simulink model "displayTest"  (R2022b)
settings: Solver=FixedStepDiscrete  StartTime=0.0  StopTime=10.0  FixedStep=0.01  RelTol=1e-3  EnableMultiTasking=on
PreLoadFcn:
  | try, model_open; catch, disp('Error occurred while executing model pre-load callback: model_open.m'); disp('Please assure that the MATLAB working directory is set to the model directory before opening.'); end
InitFcn:
  | try, model_open; catch, end
model workspace (MAT data in the model file):
  IOScreen_Label_XCoord = 1
  IOScreen_Row1_YCoord = 1
  IOScreen_Row2_YCoord = 12
  IOScreen_Value_XCoord = 110
  MainScreen_Row1_YCoord = 7
  MainScreen_Row2_YCoord = 23
  MainScreen_Symbols_XCoord = 1
  MainScreen_Units_XCoord = 69
  MainScreen_Value_XCoord = 64
undefined symbols (not defined in the file or in its folder): curr_screen, DISP, gesture, raptor_get_buildNum, raptor_get_safe_string, raptor_hwexp, raptor_xcp_function, Screens, VC500
libraries: Raptor_display_lib x93, Raptor_lib x40, Raptor_Datalogging_lib x10, simulink_extras x3, simulink x2
(part 1 of 3)
CloseFcn:
  | try, model_close; catch, end
settings Model: Raptor_Target=DISP-VC500-1904  RaptorUIDSize=4  Raptor_Calloc=NonVolatile (EEPROM)  RaptorBuildNum=0  Raptor_ecuaddr=253  Raptor_IsLiteMode=0  SimulationMode=rapid-accelerator  Creator=Ben  LastModifiedBy=Jhon
settings SolverCC: AlgebraicLoopSolver=TrustRegion
settings DataIOCC: LimitDataPoints=on  SaveFormat=Array  SignalLoggingSaveFormat=ModelDataLogs  ReturnWorkspaceOutputs=off
settings OptimizationCC: DefaultParameterBehavior=Inlined  ExpressionDepthLimit=2147483647  InitFltsAndDblsToZero=on  LifeSpan=1  EfficientTunableParamExpr=on
settings DebuggingCC: CheckSSInitialOutputMsg=off  SolverPrmCheckMsg=warning  InheritedTsInSrcMsg=none  FcnCallInpInsideContextMsg=warning  UnconnectedInputMsg=warning  UnconnectedOutputMsg=warning  UnconnectedLineMsg=warning  StateNameClashWarn=warning  PregeneratedLibrarySubsystemCodeDiagnostic=none  SFUnexpectedBacktrackingDiag=warning  SFNoUnconditionalDefaultTransitionDiag=warning  SFExecutionAtInitializationDiag=none  SFMachineParentedDataDiag=warning  ArithmeticOperatorsInVariantConditions=warning
settings HardwareCC: ProdBitPerPointer=32  ProdBitPerSizeT=32  ProdBitPerPtrDiffT=32  ProdLargestAtomicInteger=Long  ProdWordSize=32  ProdHWDeviceType=ARM Compatible->ARM 9  TargetIntDivRoundTo=Zero  TargetEndianess=BigEndian  ProdEqTarget=off
settings ModelReferenceCC: EnableRefExpFcnMdlSchedulingChecks=on  PropagateSignalLabelsOutOfModel=off
settings SFSimCC: SimUseLocalCustomCode=off  MATLABDynamicMemAlloc=off  CustomCodeUndefinedFunction=UseInterfaceOnly
settings RTWCC: Description=Raptor (tm)  SystemTargetFile=raptor.tlc  GenCodeOnly=on  MakeCommand=raptor_make_rtw  TemplateMakefile=raptor.tmf  RTWUseLocalCustomCode=off
settings CodeAppCC: IgnoreCustomStorageClasses=off  MaxIdLength=100  CustomSymbolStrType=$N$R$M  StateflowObjectComments=on  InternalIdentifier=Classic
settings STFCustomTargetCC: GenerateSampleERTMain=on  ModelReferenceCompliant=off  CombineOutputUpdateFcns=on  ERTCustomFileBanners=on  SupportContinuousTime=off  SupportNonInlinedSFcns=off  RemoveResetFunc=on  MATLABClassNameForMDSCustomization=Simulink.SoftwareTarget.ERTCustomization  SystemTargetFile=raptor.tlc
settings ERTTargetCC: MultiwordLength=2048  GenerateSampleERTMain=on  ModelReferenceCompliant=off  ParMdlRefBuildCompliant=off  CompOptLevelCompliant=off  ConcurrentExecutionCompliant=off  ModelStepFunctionPrototypeControlCompliant=off  CPPClassGenCompliant=off  UseToolchainInfoCompliant=off  ExtModeMexFile=noextcomm  InlinedParameterPlacement=NonHierarchical  ERTCustomFileTemplate=example_file_process.tlc  ConvertIfToSwitch=off  SuppressUnreachableDefaultCases=off
settings ConfigComp: CovMetricSettings=dw  CovSaveCumulativeToWorkspaceVar=on  CovSaveSingleToWorkspaceVar=on  CovExternalEMLEnable=off

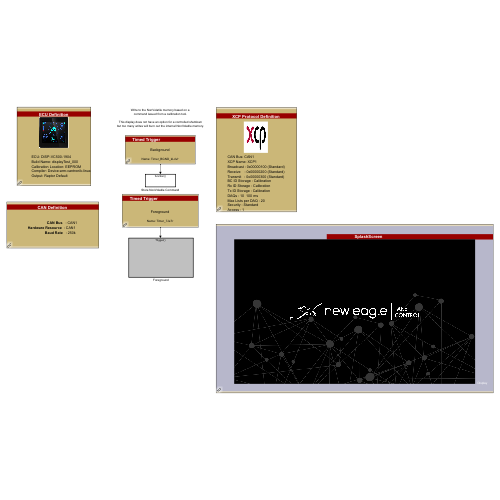
[thumbnail: Simulink's stored preview of the top-level diagram]
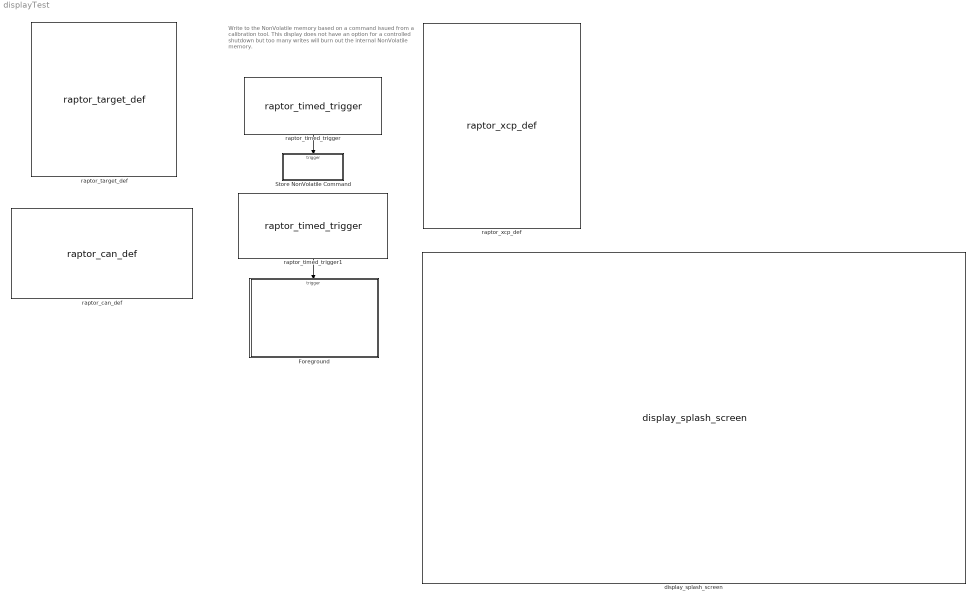
== system displayTest ==
  note: Write to the NonVolatile memory based on a
      | command issued from a calibration tool.
      |
      | This display does not have an option for a controlled shutdown
      | but too many writes will burn out the internal NonVolatile memory.
  Foreground : Subsystem
  Store NonVolatile Command : Subsystem  TreatAsAtomicUnit=on
  display_splash_screen : Raptor_display_lib/Screen Functions/display_splash_screen  ImageFile=background_newsplash.bmp
      settings: SourceProductName=Raptor Display Library
  raptor_can_def : Raptor_lib/CAN/raptor_can_def  canBus='CAN1'  resourceValues=CAN1|(None)  resource=CAN1  baudRateValues=125k|250k|500k|1000k  baudRate=250k  enable_baud_rate_config=0  sim_func_name='ConfigureCANBaudRate'  createButton=[]  txQueueSize=16  rxQueueSize=16
      settings: SourceProductName=Raptor
  raptor_target_def : Raptor_lib/Configuration/raptor_target_def  targetValues=BCM-5646-48-1404|CSM-S32K148-030-1903|DISP-VC128-1901|DISP-VC320L-1402|DISP-VC320-1204|DISP-VC800-1402|DISP-VC500-1904|DISP-VC700-2003|DISP-VC300R-2004|GCM-5634M-070-1459|GCM-5634M-070-1559|GCM-5634M-070-1562|ECM-1793-196-1503|GCM-1793-196-1503|GCM-5605B-048-1906|GCM-5607B-80-1901|GCM-5607B-80-1903|GCM-5607B-80-2001|GCM-5746R-048-1902|HCM-5534-50-1203|HCM-5534-90-1201|HCM-5534-90-1302|HCM-5534-90-1601|HCM-5534-90-1602|HCM-5604-36-1303|HCM-5604-36-1702|HCM-ARM4-070-1401|HCM-ARM4-070-1601|UAS-564A-WAL  target=DISP-VC500-1904  simpack=0  simulator=0  heap=2*1024  stack=2*1024  fgndStack=2*1024  bgndStack=2*1024  idleStack=1024  intStack=1536  sdStack=1024  appStack=1024  ecuaddr=253  uds_server_addr_ext=0  uds_server_addr=hex2dec('600')  uds_client_addr=hex2dec('650')  callocValues=Constant (FLASH)|NonVolatile (EEPROM)  calloc=NonVolatile (EEPROM)  compilerValues=Device:arm-cantronik-linux-gnueabihf_5.4.2 Simulator:None (disabled)|Device:arm-cantronik-linux-gnueabihf_5.4.2 Simulator:Visual Studio Community 2017  compiler=Device:arm-cantronik-linux-gnueabihf_5.4.2 Simulator:Visual Studio Community 2017  setFileName=1  exeName=[raptor_get_safe_string(bdroot) '_']  addBuildNum=1  minVerChars=3  extraOutput=0  buildLocationValues=Raptor Default|Model Directory|User Defined  buildLocation=Raptor Default  exeLocation=''  exeFileButton=[]  a2lLocation=''  a2lFileButton=[]  rpgLocation=''  rpgFileButton=[]
      settings: SourceProductName=Raptor
  raptor_timed_trigger : Raptor_lib/Triggers/raptor_timed_trigger  triggerValues=Foreground|Foregroundx2|Foregroundx5|Foregroundx10|Foregroundx50|Background|Backgroundx2|Backgroundx5|Backgroundx10|Backgroundx20|Second|Minute  trigger=Background  inherited=0  alwaysEnabled=1  triggerPriority=0  triggerName=BGND_kLoVr
      settings: SourceProductName=Raptor
  raptor_timed_trigger1 : Raptor_lib/Triggers/raptor_timed_trigger  triggerValues=Foreground|Foregroundx5|Foregroundx10|Foregroundx50|Second|Minute  trigger=Foreground  inherited=0  alwaysEnabled=1  triggerPriority=0  triggerName=7Je7r
      settings: SourceProductName=Raptor
  raptor_xcp_def : Raptor_lib/Configuration/raptor_xcp_def  XCPname='XCP1'  canBus='CAN1'  bcID=hex2dec('100')  bcID_TypeValues=Standard|Extended  bcID_Type=Standard  rxID=hex2dec('200')  rxID_TypeValues=Standard|Extended  rxID_Type=Standard  txID=hex2dec('300')  txID_TypeValues=Standard|Extended  txID_Type=Standard  daqRates=[10 100]  numODTs=20  genCANAPE=0  genVISION=0  securityValues=Standard|None|Custom User Defined|MH_SB_4  security=Standard  dllName=raptor_XCPSecurity.dll  accessValues=4|3|2|1  access=1  bcStorageValues=[]  bcStorage=Calibration  txStorageValues=[]  txStorage=Calibration  rxStorageValues=[]  rxStorage=Calibration
      settings: SourceProductName=Raptor
  wires:
  raptor_timed_trigger1/1 -> Foreground/Trigger
  raptor_timed_trigger/1 -> Store NonVolatile Command/Trigger

== system displayTest/Foreground ==
  Trigger : TriggerPort  TriggerType=function-call  VariantControl=Variant  PortDimensions=1
  Display : Subsystem
      mask Display: image(imread('DISP-VC500-1904.jpg'))
  Plant : Subsystem
      mask Display:
      | block = gcb;
      | pos = get_param(gcb, 'Position');
      | 
      | info = imfinfo('VeeCAN500_pinout.png');
      | 
      | pos(3) = pos(1)+info.Width;
      | pos(4) = pos(2)+info.Height;
      | 
      | set_param(block, 'Position', pos);
      | 
      | image(imread('VeeCAN500_pinout.png'));
  wires:
  Display/1(Actuators) -> Plant/1(Actuators)
  Plant/1(Sensors) -> Display/1(Sensors)

== system displayTest/Store NonVolatile Command ==
  note: Setting the StoreNonvolatileCommand value to to 1
      | in the calibration tool will cause this subsystem to execute, calling the 'Store Nonvolatile' function.
      |
      | The StoreNonvolatileCommand value will be set to 0 inside
      | the subsytem so that the Store event happens once.
  function : TriggerPort  TriggerType=function-call  VariantControl=Variant
  Store NV : Subsystem  TreatAsAtomicUnit=on
  raptor_data_def : Raptor_lib/Data Storage/raptor_data_def  dataName='StoreNonVolatileCommand'  initValue=false  dataType=boolean  storage=Volatile (RAM)  calVisible=on  calType=Adjustment  calDispType=Enumeration  calEnum={'Not Writing', 'Start Write'}  calGain=1.0  calOffset=0  calMin=-inf  calMax=inf  calFormat='-1'  calUnit=''  calHelp=''  calAccess=1  calFunction=raptor_xcp_function(gcb)  calDispHeaders=off  calColHeaders={'Col1' 'Col2' 'Col3'}  calRowHeaders={'Row1' 'Row2' 'Row3'}
      settings: SourceProductName=Raptor
  raptor_data_read : Raptor_lib/Data Storage/raptor_data_read  dataName='StoreNonVolatileCommand'  dataShape=Scalar  idxSource=Input  idxRow=1  idxCol=1
      settings: SourceProductName=Raptor
  wires:
  raptor_data_read/1 -> Store NV/Enable

== system displayTest/Foreground/Display ==
  Sensors : Inport
  Data Logging : Subsystem
  Screens : Subsystem
  Unit Delay : UnitDelay  SampleTime=-1  HasFrameUpgradeWarning=on
  Actuators : Outport  VectorParamsAs1DForOutWhenUnconnected=off
  wires:
  Sensors/1 -> Data Logging/2(Sensors), Screens/1(Sensors)
  Screens/1(ActuatorCommands) -> Actuators/1
  Screens/2(DataLogCommands) -> Data Logging/1(Commands)
  Data Logging/1(DataLogState) -> Unit Delay/1
  Unit Delay/1 -> Screens/2(DataLogState)

== system displayTest/Foreground/Plant ==
  Actuators : Inport
  Inputs : Subsystem
  Outputs : Subsystem
  Sensors : Outport  VectorParamsAs1DForOutWhenUnconnected=off
  wires:
  Actuators/1 -> Outputs/1(Commands)
  Inputs/1(Sensors) -> Sensors/1

== system displayTest/Store NonVolatile Command/Store NV ==
  Enable : EnablePort
  Constant : Constant  Value=false
  Function-Call Generator : simulink/Ports & Subsystems/Function-Call Generator  sample_time=-1  numberOfIterations=1  DisallowWideOutput=off
  raptor_data_write : Raptor_lib/Data Storage/raptor_data_write  dataName='StoreNonVolatileCommand'  dataShape=Scalar  idxSource=Input Port  idxRow=1  idxCol=1
      settings: SourceProductName=Raptor
  raptor_store_nv : Raptor_lib/Data Storage/raptor_store_nv  null=0
      settings: SourceProductName=Raptor
  wires:
  Function-Call Generator/1 -> raptor_store_nv/Trigger
  Constant/1 -> raptor_data_write/1

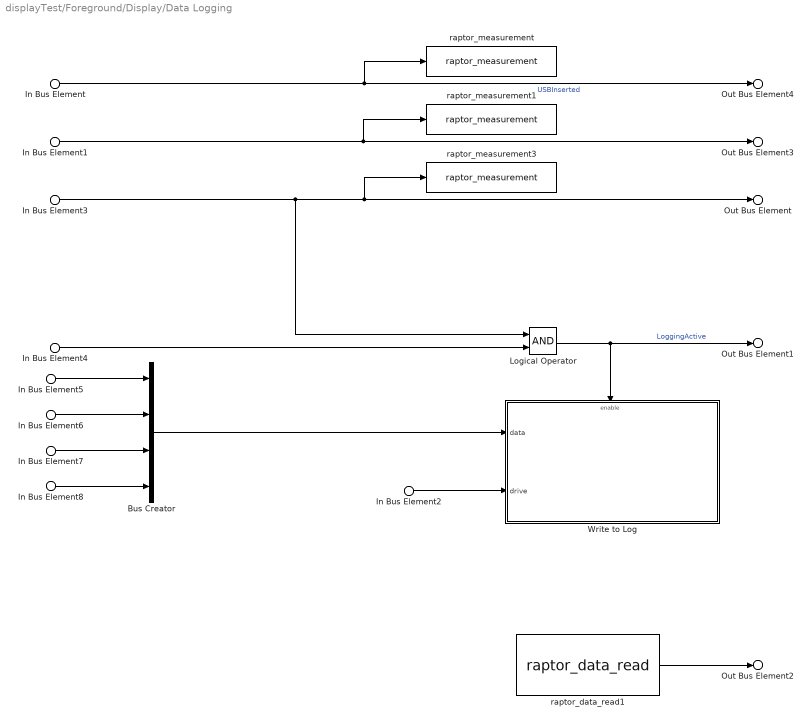
== system displayTest/Foreground/Display/Data Logging ==
  In Bus Element4 : Inport  PortName=Commands  Element=LoggingEnabled
  In Bus Element : Inport  Port=2  PortName=Sensors  Element=USBInserted
  In Bus Element1 : Inport  Port=2  PortName=Sensors  Element=USBEjectReady
  In Bus Element2 : Inport  Port=2  PortName=Sensors  Element=USBPath
  In Bus Element3 : Inport  Port=2  PortName=Sensors  Element=USBReadyToLog
  In Bus Element5 : Inport  Port=2  PortName=Sensors  Element=EngineRPM
  In Bus Element6 : Inport  Port=2  PortName=Sensors  Element=EngineRPMValid
  In Bus Element7 : Inport  Port=2  PortName=Sensors  Element=Illumination
  In Bus Element8 : Inport  Port=2  PortName=Sensors  Element=IlluminationValid
  Bus Creator : BusCreator  Inputs=4
  Logical Operator : Logic  AllPortsSameDT=off  OutDataTypeStr=boolean
  Write to Log : Subsystem
  raptor_data_read1 : Raptor_lib/Data Storage/raptor_data_read  dataName='LogCounter'  dataShape=Scalar  idxSource=Input  idxRow=1  idxCol=1
      settings: SourceProductName=Raptor
  raptor_measurement : Raptor_lib/Data Storage/raptor_measurement  paramName='USBInserted'  nameSource=Parameter  calDispType=Number  calEnum={'False', 'True'}  calGain=1.0  calOffset=0.0  calMax=inf  calMin=-inf  calFormat='-1'  calUnit=''  calHelp=''  calAccess=1  calFunction=raptor_xcp_function(gcb)  calVisible=on
      settings: SourceProductName=Raptor
  raptor_measurement1 : Raptor_lib/Data Storage/raptor_measurement  paramName='EjectReady'  nameSource=Parameter  calDispType=Number  calEnum={'False', 'True'}  calGain=1.0  calOffset=0.0  calMax=inf  calMin=-inf  calFormat='-1'  calUnit=''  calHelp=''  calAccess=1  calFunction=raptor_xcp_function(gcb)  calVisible=on
      settings: SourceProductName=Raptor
  raptor_measurement3 : Raptor_lib/Data Storage/raptor_measurement  paramName='LoggingReady'  nameSource=Parameter  calDispType=Number  calEnum={'False', 'True'}  calGain=1.0  calOffset=0.0  calMax=inf  calMin=-inf  calFormat='-1'  calUnit=''  calHelp=''  calAccess=1  calFunction=raptor_xcp_function(gcb)  calVisible=on
      settings: SourceProductName=Raptor
  Out Bus Element : Outport  VectorParamsAs1DForOutWhenUnconnected=off  PortName=DataLogState  Element=LoggingPossible
  Out Bus Element1 : Outport  VectorParamsAs1DForOutWhenUnconnected=off  PortName=DataLogState  Element=LoggingActive
  Out Bus Element2 : Outport  VectorParamsAs1DForOutWhenUnconnected=off  PortName=DataLogState  Element=LogCounter
  Out Bus Element3 : Outport  VectorParamsAs1DForOutWhenUnconnected=off  PortName=DataLogState  Element=EjectReady
  Out Bus Element4 : Outport  VectorParamsAs1DForOutWhenUnconnected=off  PortName=DataLogState  Element=USBInserted
  wires:
  In Bus Element/1 -> raptor_measurement/1, Out Bus Element4/1  "USBInserted"
  Bus Creator/1 -> Write to Log/1(data)
  In Bus Element1/1 -> raptor_measurement1/1, Out Bus Element3/1
  In Bus Element2/1 -> Write to Log/2(drive)
  In Bus Element3/1 -> raptor_measurement3/1, Out Bus Element/1, Logical Operator/1
  Logical Operator/1 -> Out Bus Element1/1, Write to Log/Enable  "LoggingActive"
  raptor_data_read1/1 -> Out Bus Element2/1
  In Bus Element4/1 -> Logical Operator/2
  In Bus Element5/1 -> Bus Creator/1
  In Bus Element6/1 -> Bus Creator/2
  In Bus Element7/1 -> Bus Creator/3
  In Bus Element8/1 -> Bus Creator/4

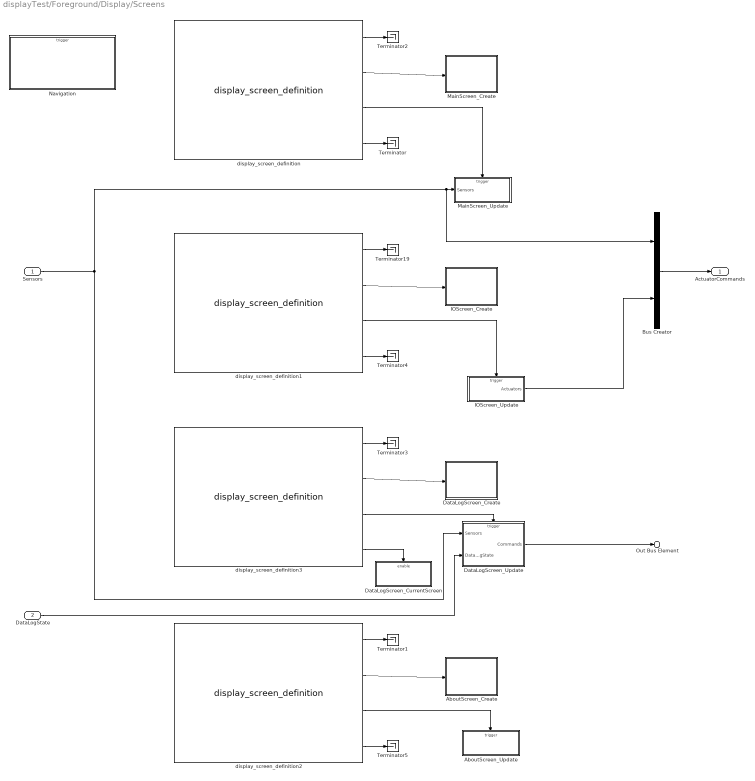
== system displayTest/Foreground/Display/Screens ==
  Sensors : Inport
  DataLogState : Inport  Port=2
  AboutScreen_Create : Subsystem  TreatAsAtomicUnit=on
  AboutScreen_Update : Subsystem  TreatAsAtomicUnit=on
  Bus Creator : BusCreator  Inputs=2
  DataLogScreen_Create : Subsystem  TreatAsAtomicUnit=on
  DataLogScreen_CurrentScreen : Subsystem  TreatAsAtomicUnit=on
  DataLogScreen_Update : Subsystem  TreatAsAtomicUnit=on
  IOScreen_Create : Subsystem  TreatAsAtomicUnit=on
  IOScreen_Update : Subsystem  TreatAsAtomicUnit=on
  MainScreen_Create : Subsystem  TreatAsAtomicUnit=on
  MainScreen_Update : Subsystem  TreatAsAtomicUnit=on
  Navigation : Subsystem
  Terminator{,1..5,19} (7 alike) : Terminator
  display_screen_definition : Raptor_display_lib/Screen Functions/display_screen_definition  ScreenName='MainScreen'  selectAtInit=true  useSimFuncs=off  useInitFunc=on  init_func_name=''  useCreateFunc=on  bgnd_func_name=''  useUpdateFunc=on  fgnd_func_name=''
      settings: SourceProductName=Raptor Display Library
  display_screen_definition1 : Raptor_display_lib/Screen Functions/display_screen_definition  ScreenName='IOScreen'  selectAtInit=false  useSimFuncs=off  useInitFunc=on  init_func_name=''  useCreateFunc=on  bgnd_func_name=''  useUpdateFunc=on  fgnd_func_name=''
      settings: SourceProductName=Raptor Display Library
  display_screen_definition2 : Raptor_display_lib/Screen Functions/display_screen_definition  ScreenName='AboutScreen'  selectAtInit=false  useSimFuncs=off  useInitFunc=on  init_func_name=''  useCreateFunc=on  bgnd_func_name=''  useUpdateFunc=on  fgnd_func_name=''
      settings: SourceProductName=Raptor Display Library
  display_screen_definition3 : Raptor_display_lib/Screen Functions/display_screen_definition  ScreenName='DataLogScreen'  selectAtInit=false  useSimFuncs=off  useInitFunc=on  init_func_name=''  useCreateFunc=on  bgnd_func_name=''  useUpdateFunc=on  fgnd_func_name=''
      settings: SourceProductName=Raptor Display Library
  ActuatorCommands : Outport  VectorParamsAs1DForOutWhenUnconnected=off
  Out Bus Element : Outport  Port=2  VectorParamsAs1DForOutWhenUnconnected=off  PortName=DataLogCommands  Element=LoggingEnabled
  wires:
  display_screen_definition/1 -> Terminator2/1
  display_screen_definition/2 -> MainScreen_Create/Trigger
  display_screen_definition/3 -> MainScreen_Update/Trigger
  display_screen_definition1/4 -> Terminator4/1
  display_screen_definition/4 -> Terminator/1
  Sensors/1 -> DataLogScreen_Update/1(Sensors), Bus Creator/1, MainScreen_Update/1(Sensors)
  display_screen_definition1/2 -> IOScreen_Create/Trigger
  display_screen_definition1/3 -> IOScreen_Update/Trigger
  display_screen_definition1/1 -> Terminator19/1
  IOScreen_Update/1(Actuators) -> Bus Creator/2
  Bus Creator/1 -> ActuatorCommands/1
  display_screen_definition2/1 -> Terminator1/1
  display_screen_definition2/3 -> AboutScreen_Update/Trigger
  display_screen_definition2/2 -> AboutScreen_Create/Trigger
  display_screen_definition2/4 -> Terminator5/1
  display_screen_definition3/4 -> DataLogScreen_CurrentScreen/Enable
  display_screen_definition3/2 -> DataLogScreen_Create/Trigger
  display_screen_definition3/3 -> DataLogScreen_Update/Trigger
  display_screen_definition3/1 -> Terminator3/1
  DataLogScreen_Update/1(Commands) -> Out Bus Element/1
  DataLogState/1 -> DataLogScreen_Update/2(DataLogState)

== system displayTest/Foreground/Plant/Inputs ==
  J1939 Rx : Subsystem
  USB : Subsystem
  Out Bus Element2 : Outport  VectorParamsAs1DForOutWhenUnconnected=off  PortName=Sensors  Element=EngineRPM
  Out Bus Element3 : Outport  VectorParamsAs1DForOutWhenUnconnected=off  PortName=Sensors  Element=EngineRPMValid
  Out Bus Element4 : Outport  VectorParamsAs1DForOutWhenUnconnected=off  PortName=Sensors  Element=Illumination
  Out Bus Element5 : Outport  VectorParamsAs1DForOutWhenUnconnected=off  PortName=Sensors  Element=IlluminationValid
  Out Bus Element1 : Outport  VectorParamsAs1DForOutWhenUnconnected=off  PortName=Sensors  Element=USBInserted
  Out Bus Element6 : Outport  VectorParamsAs1DForOutWhenUnconnected=off  PortName=Sensors  Element=USBEjectReady
  Out Bus Element7 : Outport  VectorParamsAs1DForOutWhenUnconnected=off  PortName=Sensors  Element=USBPath
  Out Bus Element8 : Outport  VectorParamsAs1DForOutWhenUnconnected=off  PortName=Sensors  Element=USBReadyToLog
  Out Bus Element9 : Outport  VectorParamsAs1DForOutWhenUnconnected=off  PortName=Sensors  Element=USBFreeSpace
  wires:
  J1939 Rx/1(Engine RPM) -> Out Bus Element2/1
  J1939 Rx/2(Engine RPM Valid) -> Out Bus Element3/1
  J1939 Rx/3(Illumination) -> Out Bus Element4/1
  J1939 Rx/4(Illumination1) -> Out Bus Element5/1
  USB/1(USBInserted) -> Out Bus Element1/1
  USB/2(USBEjectReady) -> Out Bus Element6/1
  USB/3(USBPath) -> Out Bus Element7/1
  USB/4(USBReadyToLog) -> Out Bus Element8/1
  USB/5(USBFreeSpace) -> Out Bus Element9/1

== system displayTest/Foreground/Plant/Outputs ==
  In Bus Element : Inport  PortName=Commands  Element=signal1.Illumination
  In Bus Element2 : Inport  PortName=Commands  Element=signal2.Buzzer
  In Bus Element3 : Inport  PortName=Commands  Element=signal2.BuzzerMute
  Constant : Constant  OutDataTypeStr=uint32
  Data Type Conversion : DataTypeConversion  OutDataTypeStr=uint16  SaturateOnIntegerOverflow=off  RndMeth=Floor
  Gain : Gain  Gain=100  OutDataTypeStr=single  RndMeth=Simplest  SaturateOnIntegerOverflow=on
  raptor_digital_out6 : Raptor_lib/Input & Output/raptor_digital_out  resourceValues=OUTPUT1|BUZZER_MUTE|BUZZER|(None)  resource=BUZZER_MUTE  driverTypeValues=Internal  driverType=Internal
      settings: SourceProductName=Raptor
  raptor_digital_out7 : Raptor_lib/Input & Output/raptor_digital_out  resourceValues=OUTPUT1|BUZZER_MUTE|BUZZER|(None)  resource=BUZZER  driverTypeValues=Internal  driverType=Internal
      settings: SourceProductName=Raptor
  raptor_pwm_out : Raptor_lib/Input & Output/raptor_pwm_out  showEnable=0  resourceValues=OUTPUT1|LED1|LED2|LED3|LED4|LCD_BACKLIGHT|KEYPAD_BACKLIGHT|(None)  resource=LCD_BACKLIGHT  driverTypeValues=LED  driverType=LED
      settings: SourceProductName=Raptor
  wires:
  In Bus Element/1 -> Gain/1
  Gain/1 -> Data Type Conversion/1
  Data Type Conversion/1 -> raptor_pwm_out/1
  Constant/1 -> raptor_pwm_out/2
  In Bus Element2/1 -> raptor_digital_out7/1
  In Bus Element3/1 -> raptor_digital_out6/1

== system displayTest/Foreground/Display/Data Logging/Write to Log ==
  data : Inport
  drive : Inport  Port=2
  Enable : EnablePort
  Create New File : Subsystem  TreatAsAtomicUnit=on
  File Write Action : Subsystem
  If : If  IfExpression=u1
  Merge : Merge
  Merge1 : Merge
  Open Existing File : Subsystem  TreatAsAtomicUnit=on
  raptor_fileIO_exists1 : Raptor_Datalogging_lib/raptor_fileIO_exists  resourceValues=Data|USB|(None)  resource=USB
      settings: SourceProductName=Raptor Data Logging
  raptor_measurement1 : Raptor_lib/Data Storage/raptor_measurement  paramName='FileOpen_Success'  nameSource=Parameter  calDispType=Number  calEnum={'False', 'True'}  calGain=1.0  calOffset=0.0  calMax=inf  calMin=-inf  calFormat='4.2'  calUnit=''  calHelp=''  calAccess=4  calFunction=raptor_xcp_function(gcb)  calVisible=on
      settings: SourceProductName=Raptor
  raptor_string1 : Raptor_lib/Strings/raptor_string  stringName='LogFileName'  string=''  dynamicSize=Fixed Size  strSize=125  storage=Volatile (RAM)  calVisible=on  calAccess=4  strFunction=raptor_xcp_function(gcb)
      settings: SourceProductName=Raptor
  raptor_string_printf : Raptor_lib/Strings/raptor_string_printf  formatString='%s/log.txt'
      settings: SourceProductName=Raptor
  wires:
  drive/1 -> raptor_string_printf/2
  Merge1/1 -> raptor_measurement1/1, File Write Action/Enable
  raptor_string1/1 -> raptor_string_printf/1
  raptor_string_printf/1 -> raptor_fileIO_exists1/1, Create New File/1(Path), Open Existing File/1(Path)
  raptor_fileIO_exists1/1 -> If/1
  If/1 -> Open Existing File/Action
  If/2 -> Create New File/Action
  Open Existing File/1(Handle) -> Merge/1
  Create New File/1(Handle) -> Merge/2
  Open Existing File/2(Sucess) -> Merge1/1
  Create New File/2(Success) -> Merge1/2
  data/1 -> File Write Action/1(data)
  Merge/1 -> File Write Action/2(In2)

== system displayTest/Foreground/Display/Screens/AboutScreen_Create ==
  function : TriggerPort  TriggerType=function-call  VariantControl=Variant
  AboutScreenSwipe : Subsystem
  Constant16 : Constant  Value=400  OutDataTypeStr=int32
  Constant2 : Constant  Value=440  OutDataTypeStr=int32
  Constant3 : Constant  OutDataTypeStr=int32
  Constant4 : Constant  OutDataTypeStr=int32
  Constant5 : Constant  OutDataTypeStr=int32
  Constant6 : Constant  Value=207  OutDataTypeStr=int32
  display_clear_screen : Raptor_display_lib/Drawing Functions/display_clear_screen  Priority=100  colorPort=off  l1Color=0000  l2Color=FFFF  pnPort=off
      settings: SourceProductName=Raptor Display Library
  display_draw_image : Raptor_display_lib/Drawing Functions/display_draw_image  imagePort=off  imageFile=top corner logo.png  opacityPort=off  opacity=100  drawMode=Draw Entire Image  alpha=Draw as Transparent  layer=Background  drawModeXY=Top Left  pnPort=off
      settings: SourceProductName=Raptor Display Library
  display_draw_image1 : Raptor_display_lib/Drawing Functions/display_draw_image  imagePort=off  imageFile=swipe_right_left.png  opacityPort=off  opacity=100  drawMode=Draw Entire Image  alpha=Draw as Transparent  layer=Foreground  drawModeXY=Top Left  pnPort=off
      settings: SourceProductName=Raptor Display Library
  display_draw_text : Raptor_display_lib/Drawing Functions/display_draw_text  textPort=off  textVal='About'  colorPort=off  col=FFFF  opacity=100  font=Future  fontFile=''  heightPort=off  height=40  hAlign=Center  vAlign=Center  spacing=0  layer=Background  pnPort=off
      settings: SourceProductName=Raptor Display Library
  raptor_display_swipe_action2 : Raptor_display_lib/Touchscreen/raptor_display_swipe_action  gest_callback_sim_func_name='AboutScreenSwipe'
      settings: SourceProductName=Raptor Display Library
  wires:
  Constant16/1 -> display_draw_text/1
  Constant2/1 -> display_draw_text/2
  Constant4/1 -> display_draw_image/1
  Constant3/1 -> display_draw_image/2
  Constant6/1 -> display_draw_image1/1
  Constant5/1 -> display_draw_image1/2

== system displayTest/Foreground/Display/Screens/AboutScreen_Update ==
  function : TriggerPort  TriggerType=function-call  VariantControl=Variant
  AboutElement : Subsystem
  display_element1 : Raptor_display_lib/Drawing Functions/display_element  colorPort=off  col=0000  layer=Background  pnPort=off
      settings: SourceProductName=Raptor Display Library
  wires:
  display_element1/1 -> AboutElement/Trigger

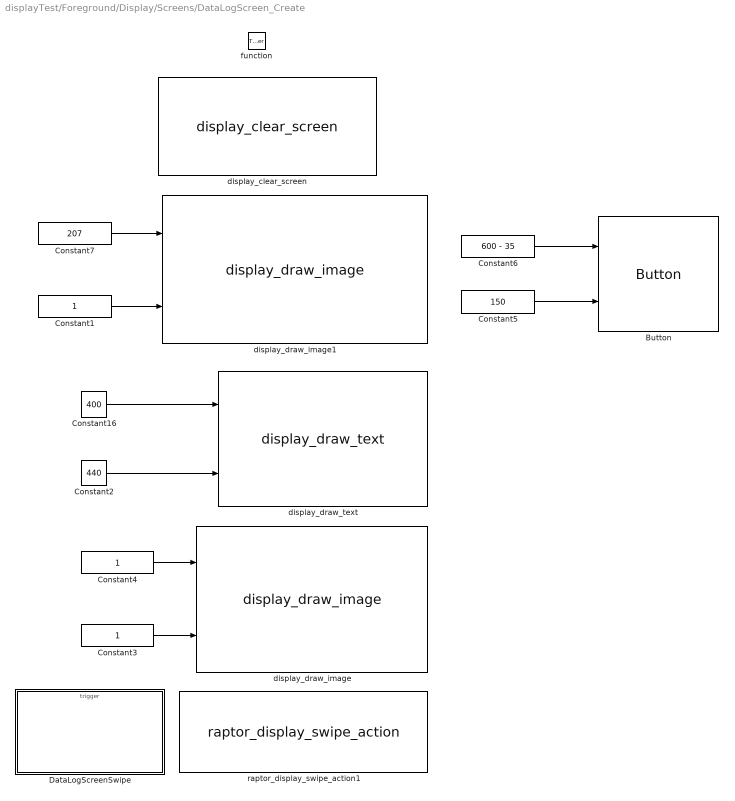
== system displayTest/Foreground/Display/Screens/DataLogScreen_Create ==
  function : TriggerPort  TriggerType=function-call  VariantControl=Variant
  Button : Raptor_display_lib/Prefab/Button  ButtonName='EjectButtonScreen'  ImageFile='eject_button.png'  PressedImageFile='eject_button_pressed.png'  font=Arial  fontFile=''  TextLine1=''  HeightLine1=12  TextLine2=''  HeightLine2=12  TextUnderButton=''  HeightUnderButton=12  buttonMargin=0  underMargin=0  buttonVAlign=Center  underVAlign=Center  buttonHAlign=Center  underHAlign=Center  underSide=Bottom  col='0000'  pressedCol='07E0'  underCol='0000'  pressedUnderCol='07E0'
      settings: SourceProductName=Raptor Display Library
  Constant1 : Constant  OutDataTypeStr=int32
  Constant16 : Constant  Value=400  OutDataTypeStr=int32
  Constant2 : Constant  Value=440  OutDataTypeStr=int32
  Constant3 : Constant  OutDataTypeStr=int32
  Constant4 : Constant  OutDataTypeStr=int32
  Constant5 : Constant  Value=150  OutDataTypeStr=int32
  Constant6 : Constant  Value=600 - 35  OutDataTypeStr=int32
  Constant7 : Constant  Value=207  OutDataTypeStr=int32
  DataLogScreenSwipe : Subsystem
  display_clear_screen : Raptor_display_lib/Drawing Functions/display_clear_screen  Priority=100  colorPort=off  l1Color=0000  l2Color=FFFF  pnPort=off
      settings: SourceProductName=Raptor Display Library
  display_draw_image : Raptor_display_lib/Drawing Functions/display_draw_image  imagePort=off  imageFile=top corner logo.png  opacityPort=off  opacity=100  drawMode=Draw Entire Image  alpha=Draw as Transparent  layer=Background  drawModeXY=Top Left  pnPort=off
      settings: SourceProductName=Raptor Display Library
  display_draw_image1 : Raptor_display_lib/Drawing Functions/display_draw_image  imagePort=off  imageFile=swipe_right_left.png  opacityPort=off  opacity=100  drawMode=Draw Entire Image  alpha=Draw as Transparent  layer=Foreground  drawModeXY=Top Left  pnPort=off
      settings: SourceProductName=Raptor Display Library
  display_draw_text : Raptor_display_lib/Drawing Functions/display_draw_text  textPort=off  textVal='Data Logging'  colorPort=off  col=FFFF  opacity=100  font=Future  fontFile=''  heightPort=off  height=40  hAlign=Center  vAlign=Center  spacing=0  layer=Background  pnPort=off
      settings: SourceProductName=Raptor Display Library
  raptor_display_swipe_action1 : Raptor_display_lib/Touchscreen/raptor_display_swipe_action  gest_callback_sim_func_name='DataLogScreenSwipe'
      settings: SourceProductName=Raptor Display Library
  wires:
  Constant3/1 -> display_draw_image/2
  Constant4/1 -> display_draw_image/1
  Constant2/1 -> display_draw_text/2
  Constant16/1 -> display_draw_text/1
  Constant5/1 -> Button/2
  Constant6/1 -> Button/1
  Constant7/1 -> display_draw_image1/1
  Constant1/1 -> display_draw_image1/2

== system displayTest/Foreground/Display/Screens/DataLogScreen_CurrentScreen ==
  Enable : EnablePort
  Display Button Status1 : Raptor_display_lib/Touchscreen/Display Button Status  ButtonName='EjectButtonScreen'
      settings: SourceProductName=Raptor Display Library
  EjectButtonPressed : Subsystem
  wires:
  Display Button Status1/1 -> EjectButtonPressed/Trigger

== system displayTest/Foreground/Display/Screens/DataLogScreen_Update ==
  Sensors : Inport
  DataLogState : Inport  Port=2
  function : TriggerPort  TriggerType=function-call  VariantControl=Variant
  Element : Subsystem
  display_element1 : Raptor_display_lib/Drawing Functions/display_element  colorPort=off  col=0000  layer=Background  pnPort=off
      settings: SourceProductName=Raptor Display Library
  Commands : Outport  VectorParamsAs1DForOutWhenUnconnected=off
  wires:
  display_element1/1 -> Element/Trigger
  Element/1(LoggingEnabled) -> Commands/1
  DataLogState/1 -> Element/1(DataLogState)
  Sensors/1 -> Element/2(Sensors)

== system displayTest/Foreground/Display/Screens/IOScreen_Create ==
  function : TriggerPort  TriggerType=function-call  VariantControl=Variant
  Constant16 : Constant  Value=400  OutDataTypeStr=int32
  Constant2 : Constant  Value=440  OutDataTypeStr=int32
  Constant3 : Constant  OutDataTypeStr=int32
  Constant4 : Constant  OutDataTypeStr=int32
  Constant5 : Constant  OutDataTypeStr=int32
  Constant6 : Constant  Value=207  OutDataTypeStr=int32
  IOScreenSwipe : Subsystem
  display_clear_screen : Raptor_display_lib/Drawing Functions/display_clear_screen  Priority=100  colorPort=off  l1Color=0000  l2Color=FFFF  pnPort=off
      settings: SourceProductName=Raptor Display Library
  display_draw_image : Raptor_display_lib/Drawing Functions/display_draw_image  imagePort=off  imageFile=top corner logo.png  opacityPort=off  opacity=100  drawMode=Draw Entire Image  alpha=Draw as Transparent  layer=Background  drawModeXY=Top Left  pnPort=off
      settings: SourceProductName=Raptor Display Library
  display_draw_image1 : Raptor_display_lib/Drawing Functions/display_draw_image  imagePort=off  imageFile=swipe_right_left.png  opacityPort=off  opacity=100  drawMode=Draw Entire Image  alpha=Draw as Transparent  layer=Foreground  drawModeXY=Top Left  pnPort=off
      settings: SourceProductName=Raptor Display Library
  display_draw_text : Raptor_display_lib/Drawing Functions/display_draw_text  textPort=off  textVal='I / O'  colorPort=off  col=FFFF  opacity=100  font=Future  fontFile=''  heightPort=off  height=40  hAlign=Center  vAlign=Center  spacing=0  layer=Background  pnPort=off
      settings: SourceProductName=Raptor Display Library
  raptor_display_swipe_action2 : Raptor_display_lib/Touchscreen/raptor_display_swipe_action  gest_callback_sim_func_name='IOScreenSwipe'
      settings: SourceProductName=Raptor Display Library
  wires:
  Constant2/1 -> display_draw_text/2
  Constant16/1 -> display_draw_text/1
  Constant4/1 -> display_draw_image/1
  Constant3/1 -> display_draw_image/2
  Constant5/1 -> display_draw_image1/2
  Constant6/1 -> display_draw_image1/1

== system displayTest/Foreground/Display/Screens/IOScreen_Update ==
  function : TriggerPort  TriggerType=function-call  VariantControl=Variant
  IOElement1 : Subsystem
  display_element1 : Raptor_display_lib/Drawing Functions/display_element  colorPort=off  col=0000  layer=Background  pnPort=off
      settings: SourceProductName=Raptor Display Library
  Actuators : Outport  VectorParamsAs1DForOutWhenUnconnected=off
  wires:
  IOElement1/1(Actuators) -> Actuators/1
  display_element1/1 -> IOElement1/Trigger

== system displayTest/Foreground/Display/Screens/MainScreen_Create ==
  function : TriggerPort  TriggerType=function-call  VariantControl=Variant
  Constant16 : Constant  Value=400  OutDataTypeStr=int32
  Constant2 : Constant  Value=440  OutDataTypeStr=int32
  Constant3 : Constant  OutDataTypeStr=int32
  Constant4 : Constant  OutDataTypeStr=int32
  Constant5 : Constant  OutDataTypeStr=int32
  Constant6 : Constant  Value=207  OutDataTypeStr=int32
  MainScreenSwipe : Subsystem
  display_clear_screen : Raptor_display_lib/Drawing Functions/display_clear_screen  Priority=100  colorPort=off  l1Color=0000  l2Color=FFFF  pnPort=off
      settings: SourceProductName=Raptor Display Library
  display_draw_image : Raptor_display_lib/Drawing Functions/display_draw_image  imagePort=off  imageFile=top corner logo.png  opacityPort=off  opacity=100  drawMode=Draw Entire Image  alpha=Draw as Transparent  layer=Background  drawModeXY=Top Left  pnPort=off
      settings: SourceProductName=Raptor Display Library
  display_draw_image1 : Raptor_display_lib/Drawing Functions/display_draw_image  imagePort=off  imageFile=swipe_right_left.png  opacityPort=off  opacity=100  drawMode=Draw Entire Image  alpha=Draw as Transparent  layer=Foreground  drawModeXY=Top Left  pnPort=off
      settings: SourceProductName=Raptor Display Library
  display_draw_text : Raptor_display_lib/Drawing Functions/display_draw_text  textPort=off  textVal='J1939'  colorPort=off  col=FFFF  opacity=100  font=Future  fontFile=''  heightPort=off  height=40  hAlign=Center  vAlign=Center  spacing=0  layer=Background  pnPort=off
      settings: SourceProductName=Raptor Display Library
  raptor_display_swipe_action1 : Raptor_display_lib/Touchscreen/raptor_display_swipe_action  gest_callback_sim_func_name='MainScreenSwipe'
      settings: SourceProductName=Raptor Display Library
  wires:
  Constant2/1 -> display_draw_text/2
  Constant16/1 -> display_draw_text/1
  Constant4/1 -> display_draw_image/1
  Constant3/1 -> display_draw_image/2
  Constant6/1 -> display_draw_image1/1
  Constant5/1 -> display_draw_image1/2

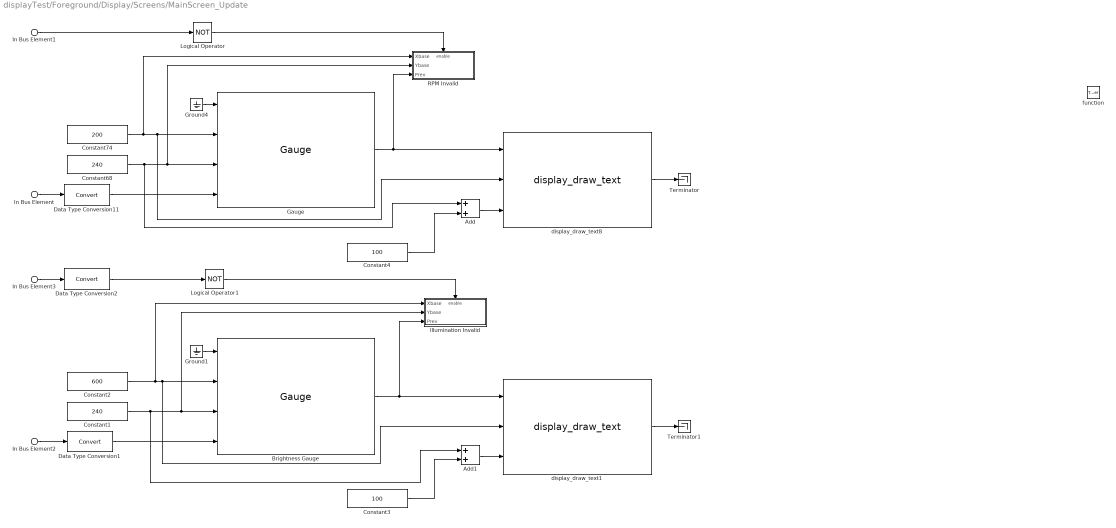
== system displayTest/Foreground/Display/Screens/MainScreen_Update ==
  In Bus Element : Inport  PortName=Sensors  Element=EngineRPM
  In Bus Element1 : Inport  PortName=Sensors  Element=EngineRPMValid
  In Bus Element2 : Inport  PortName=Sensors  Element=Illumination
  In Bus Element3 : Inport  PortName=Sensors  Element=IlluminationValid
  function : TriggerPort  TriggerType=function-call  VariantControl=Variant
  Add : Sum
  Add1 : Sum
  Brightness Gauge : Raptor_display_lib/Prefab/Gauge  Min=0  Max=100  ScaleValue=1  Dir=Clockwise  StartAngle=-135  StopAngle=135  Scale=150  GaugeFontSize=15  LargeMark=5  SmallMark=2  ArcEnable=off  NeedleColor=EF7D  MarkerColor=FFFF  Image=mgaugeBlk.bmp  imageXOffset=0  imageYOffset=0
      settings: SourceProductName=Raptor Display Library
  Constant1 : Constant  Value=240  OutDataTypeStr=int32
  Constant2 : Constant  Value=600  OutDataTypeStr=int32
  Constant3 : Constant  Value=100  OutDataTypeStr=int32
  Constant4 : Constant  Value=100  OutDataTypeStr=int32
  Constant68 : Constant  Value=240  OutDataTypeStr=int32
  Constant74 : Constant  Value=200  OutDataTypeStr=int32
  Data Type Conversion1 : DataTypeConversion  SaturateOnIntegerOverflow=off  RndMeth=Floor
  Data Type Conversion11 : DataTypeConversion  SaturateOnIntegerOverflow=off  RndMeth=Floor
  Data Type Conversion2 : DataTypeConversion  SaturateOnIntegerOverflow=off  RndMeth=Floor
  Gauge : Raptor_display_lib/Prefab/Gauge  Min=0  Max=8000  ScaleValue=1  Dir=Clockwise  StartAngle=-135  StopAngle=135  Scale=150  GaugeFontSize=15  LargeMark=5  SmallMark=2  ArcEnable=off  NeedleColor=EF7D  MarkerColor=FFFF  Image=mgaugeBlk.bmp  imageXOffset=0  imageYOffset=0
      settings: SourceProductName=Raptor Display Library
  Ground1 : Ground
  Ground4 : Ground
  Illumination Invalid : Subsystem  TreatAsAtomicUnit=on
  Logical Operator : Logic  Operator=NOT  AllPortsSameDT=off  OutDataTypeStr=boolean
  Logical Operator1 : Logic  Operator=NOT  AllPortsSameDT=off  OutDataTypeStr=boolean
  RPM Invalid : Subsystem  TreatAsAtomicUnit=on
  Terminator : Terminator
  Terminator1 : Terminator
  display_draw_text1 : Raptor_display_lib/Drawing Functions/display_draw_text  textPort=off  textVal='Brightness'  colorPort=off  col=FFFF  opacity=100  font=Future  fontFile=''  heightPort=off  height=20  hAlign=Center  vAlign=Center  spacing=0  layer=Background  pnPort=on
      settings: SourceProductName=Raptor Display Library
  display_draw_text8 : Raptor_display_lib/Drawing Functions/display_draw_text  textPort=off  textVal='RPM'  colorPort=off  col=FFFF  opacity=100  font=Future  fontFile=''  heightPort=off  height=20  hAlign=Center  vAlign=Center  spacing=0  layer=Background  pnPort=on
      settings: SourceProductName=Raptor Display Library
  wires:
  Constant68/1 -> Add/1, RPM Invalid/2(Ybase), Gauge/3
  In Bus Element/1 -> Data Type Conversion11/1
  Data Type Conversion11/1 -> Gauge/4
  Ground4/1 -> Gauge/1
  Gauge/1 -> RPM Invalid/3(Prev), display_draw_text8/1
  Ground1/1 -> Brightness Gauge/1
  Data Type Conversion1/1 -> Brightness Gauge/4
  In Bus Element2/1 -> Data Type Conversion1/1
  In Bus Element1/1 -> Logical Operator/1
  Logical Operator/1 -> RPM Invalid/Enable
  Logical Operator1/1 -> Illumination Invalid/Enable
  In Bus Element3/1 -> Data Type Conversion2/1
  Data Type Conversion2/1 -> Logical Operator1/1
  display_draw_text8/1 -> Terminator/1
  Constant74/1 -> RPM Invalid/1(Xbase), display_draw_text8/2, Gauge/2
  Constant4/1 -> Add/2
  Add/1 -> display_draw_text8/3
  Add1/1 -> display_draw_text1/3
  Constant3/1 -> Add1/2
  Constant2/1 -> Illumination Invalid/1(Xbase), display_draw_text1/2, Brightness Gauge/2
  display_draw_text1/1 -> Terminator1/1
  Brightness Gauge/1 -> display_draw_text1/1, Illumination Invalid/3(Prev)
  Constant1/1 -> Add1/1, Illumination Invalid/2(Ybase), Brightness Gauge/3

== system displayTest/Foreground/Display/Screens/Navigation ==
  Navigation : TriggerPort  TriggerType=function-call  IsSimulinkFunction=on  FunctionName=Navigation  FunctionVisibility=scoped  VariantControl=Variant  PortDimensions=1
  Go Left : Subsystem  TreatAsAtomicUnit=on
  Go Right : Subsystem  TreatAsAtomicUnit=on
  Go Up or Down : Subsystem  TreatAsAtomicUnit=on
  If : If  IfExpression=u1 == 3  ElseIfExpressions=u1 == 2
  gesture : ArgIn  OutDataTypeStr=uint8  ArgumentName=gesture
  curr_screen : ArgIn  Port=2  OutDataTypeStr=uint8  ArgumentName=curr_screen
  wires:
  gesture/1 -> If/1
  curr_screen/1 -> Go Right/1(Current Screen), Go Left/1(Current Screen), Go Up or Down/1(Current Screen)
  If/1 -> Go Right/Action
  If/2 -> Go Left/Action
  If/3 -> Go Up or Down/Action

== system displayTest/Foreground/Plant/Inputs/J1939 Rx ==
  Process Illumination Message : Subsystem
  Process RPM Message : Subsystem
  raptor_can_rxmsg : Raptor_lib/CAN/raptor_can_rxmsg  canDefinition=struct('dbcFile', 'j1939_small.dbc','message', 'CL','comment', '','signals', {{'IlluminationBrightnessPercent'}},'enabled', [ 1;],'canBus', '''CAN1''','messageID', [ 416349696;],'idMask', [ 536870656;],'payloadMask', [],'payloadValue', [],'period', [ 0;],'mailbox', '''''','queueSize', [ 1;],'label', [ 0;],'ver', [ 2;],'showID', [ 0;],'showRaw', [ 0;],'fill', [ 0;],'editID', [ 1;],'signalOrder', [ 1;])  canBus='CAN1'  mailbox=''  payloadMask=[]  payloadValue=[]  idMask=hex2dec('1FFFFF00')  queueSize=1  showID=0  label=0  fill=0  id=416349696  showRaw=0  showAge=1  signalOrder=1  signalInfo={{struct('Name', 'IlluminationBrightnessPercent','StartBit', [ 0;],'SignalSize', [ 8;],'ByteOrder', 'LittleEndian','ValueType', 'UNSIGNED','Class', 'uint8','Signed', [ 0;],'Factor', [ 0.4;],'Offset', [ 0;],'Min', [ 0;],'Max', [ 100;],'Units', '%','StartVal', [ 0;],'Comment', 'Commanded backlight brightness level for all cab displays','Multiplexed', [ 0;],'Multiplexor', [ 0;],'MultiplexMode_Min', [ 0;],'MultiplexMode_Max', [ 0;])}}  showRawMsg=0  useSimFunc=0  sim_func_name=''  useStartVals=0  extendedId=1
      settings: SourceProductName=Raptor
  raptor_can_rxmsg1 : Raptor_lib/CAN/raptor_can_rxmsg  canDefinition=struct('dbcFile', 'j1939_small.dbc','message', 'EEC1','comment', '','signals', {{'EngSpeed'}},'enabled', [ 1;],'canBus', '''CAN1''','messageID', [ 217056256;],'idMask', [ 536870656;],'payloadMask', [],'payloadValue', [],'period', [ 0;],'mailbox', '''''','queueSize', [ 1;],'label', [ 0;],'ver', [ 2;],'showID', [ 0;],'showRaw', [ 0;],'fill', [ 0;],'editID', [ 1;],'signalOrder', [ 1;])  canBus='CAN1'  mailbox=''  payloadMask=[]  payloadValue=[]  idMask=hex2dec('1FFFFF00')  queueSize=1  showID=0  label=0  fill=0  id=217056256  showRaw=0  showAge=1  signalOrder=1  signalInfo={{struct('Name', 'EngSpeed','StartBit', [ 24;],'SignalSize', [ 16;],'ByteOrder', 'LittleEndian','ValueType', 'UNSIGNED','Class', 'uint16','Signed', [ 0;],'Factor', [ 0.125;],'Offset', [ 0;],'Min', [ 0;],'Max', [ 8031.88;],'Units', 'rpm','StartVal', [ 0;],'Comment', 'Actual engine speed which is calculated over a minimum crankshaft angle of 720 degrees divided by the number of cylinders.','Multiplexed', [ 0;],'Multiplexor', [ 0;],'MultiplexMode_Min', [ 0;],'MultiplexMode_Max', [ 0;])}}  showRawMsg=0  useSimFunc=0  sim_func_name=''  useStartVals=0  extendedId=1
      settings: SourceProductName=Raptor
  Engine RPM : Outport  VectorParamsAs1DForOutWhenUnconnected=off
  Engine RPM Valid : Outport  Port=2  VectorParamsAs1DForOutWhenUnconnected=off
  Illumination : Outport  Port=3  VectorParamsAs1DForOutWhenUnconnected=off
  Illumination1 : Outport  Port=4  VectorParamsAs1DForOutWhenUnconnected=off
  wires:
  Process RPM Message/1(EngineRPM) -> Engine RPM/1
  Process Illumination Message/1(Illumination) -> Illumination/1
  Process RPM Message/2(EngineRPMValid) -> Engine RPM Valid/1
  raptor_can_rxmsg1/1 -> Process RPM Message/1(AgeCount)
  raptor_can_rxmsg1/2 -> Process RPM Message/2(Data)
  raptor_can_rxmsg/1 -> Process Illumination Message/1(AgeCount)
  raptor_can_rxmsg/2 -> Process Illumination Message/2(Data)
  Process Illumination Message/2(IlluminationValid) -> Illumination1/1

== system displayTest/Foreground/Plant/Inputs/USB ==
  raptor_fileIO_USBStatus : Raptor_Datalogging_lib/raptor_fileIO_USBStatus  showInserted=on  showEjectReady=on  showPath=on  showReadyToLog=on
      settings: SourceProductName=Raptor Data Logging
  raptor_fileIO_getFreeSpace : Raptor_Datalogging_lib/raptor_fileIO_getFreeSpace  resourceValues=USB|(None)  resource=USB
      settings: SourceProductName=Raptor Data Logging
  raptor_string : Raptor_lib/Strings/raptor_string  stringName=''  string=''  dynamicSize=Fixed Size  strSize=20  storage=Volatile (RAM)  calVisible=off  calAccess=4  strFunction=raptor_xcp_function(gcb)
      settings: SourceProductName=Raptor
  USBInserted : Outport  VectorParamsAs1DForOutWhenUnconnected=off
  USBEjectReady : Outport  Port=2  VectorParamsAs1DForOutWhenUnconnected=off
  USBPath : Outport  Port=3  VectorParamsAs1DForOutWhenUnconnected=off
  USBReadyToLog : Outport  Port=4  VectorParamsAs1DForOutWhenUnconnected=off
  USBFreeSpace : Outport  Port=5  VectorParamsAs1DForOutWhenUnconnected=off
  wires:
  raptor_fileIO_USBStatus/1 -> USBInserted/1
  raptor_fileIO_USBStatus/4 -> USBReadyToLog/1
  raptor_fileIO_USBStatus/3 -> USBPath/1
  raptor_fileIO_USBStatus/2 -> USBEjectReady/1
  raptor_string/1 -> raptor_fileIO_USBStatus/1
  raptor_fileIO_getFreeSpace/1 -> USBFreeSpace/1

== system displayTest/Foreground/Display/Data Logging/Write to Log/Create New File ==
  Path : Inport
  Action Port : ActionPort  ActionPortLabel=else
  raptor_fileIO_open1 : Raptor_Datalogging_lib/raptor_fileIO_open  resourceValues=USB|(None)  resource=USB  modeValues=Read Only|Write Only - Overwrite|Read/Write - Update|Read/Write - Overwrite  mode=2
      settings: SourceProductName=Raptor Data Logging
  Handle : Outport  VectorParamsAs1DForOutWhenUnconnected=off
  Success : Outport  Port=2  VectorParamsAs1DForOutWhenUnconnected=off
  wires:
  Path/1 -> raptor_fileIO_open1/1
  raptor_fileIO_open1/1 -> Handle/1
  raptor_fileIO_open1/2 -> Success/1

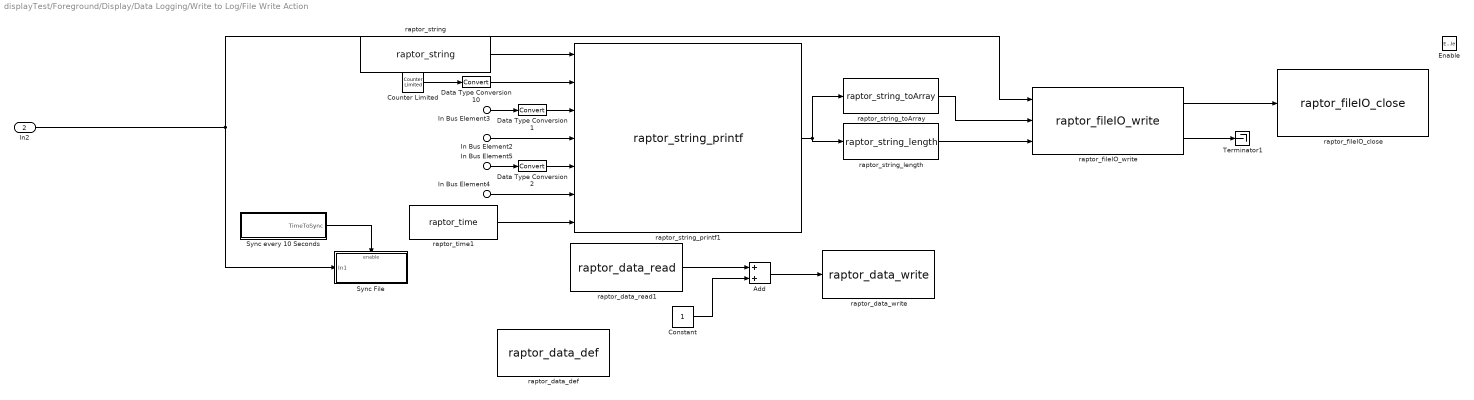
== system displayTest/Foreground/Display/Data Logging/Write to Log/File Write Action ==
  In Bus Element2 : Inport  PortName=data  Element=EngineRPM
  In Bus Element3 : Inport  PortName=data  Element=EngineRPMValid
  In Bus Element4 : Inport  PortName=data  Element=Illumination
  In Bus Element5 : Inport  PortName=data  Element=IlluminationValid
  In2 : Inport  Port=2
  Enable : EnablePort
  Add : Sum
  Constant : Constant  OutDataTypeStr=uint32
  Counter Limited : simulink/Sources/Counter Limited  uplimit=65535  tsamp=-1
  Data Type Conversion1 : DataTypeConversion  SaturateOnIntegerOverflow=off  RndMeth=Floor
  Data Type Conversion10 : DataTypeConversion  SaturateOnIntegerOverflow=off  RndMeth=Floor
  Data Type Conversion2 : DataTypeConversion  SaturateOnIntegerOverflow=off  RndMeth=Floor
  Sync File : Subsystem  TreatAsAtomicUnit=on
  Sync every 10 Seconds : Subsystem
  Terminator1 : Terminator
  raptor_data_def : Raptor_lib/Data Storage/raptor_data_def  dataName='LogCounter'  initValue=0  dataType=uint32  storage=Volatile (RAM)  calVisible=on  calType=Measurement  calDispType=Number  calEnum={'False', 'True'}  calGain=1.0  calOffset=0  calMin=-inf  calMax=inf  calFormat='-1'  calUnit=''  calHelp=''  calAccess=1  calFunction=raptor_xcp_function(gcb)  calDispHeaders=off  calColHeaders={'Col1' 'Col2' 'Col3'}  calRowHeaders={'Row1' 'Row2' 'Row3'}
      settings: SourceProductName=Raptor
  raptor_data_read1 : Raptor_lib/Data Storage/raptor_data_read  dataName='LogCounter'  dataShape=Scalar  idxSource=Input  idxRow=1  idxCol=1
      settings: SourceProductName=Raptor
  raptor_data_write : Raptor_lib/Data Storage/raptor_data_write  dataName='LogCounter'  dataShape=Scalar  idxSource=Input Port  idxRow=1  idxCol=1
      settings: SourceProductName=Raptor
  raptor_fileIO_close : Raptor_Datalogging_lib/raptor_fileIO_close  resourceValues=USB|(None)  resource=USB
      settings: SourceProductName=Raptor Data Logging
  raptor_fileIO_write : Raptor_Datalogging_lib/raptor_fileIO_write  resourceValues=Data|USB|(None)  resource=USB
      settings: SourceProductName=Raptor Data Logging
  raptor_string : Raptor_lib/Strings/raptor_string  stringName=''  string=''  dynamicSize=Fixed Size  strSize=100  storage=Volatile (RAM)  calVisible=on  calAccess=4  strFunction=raptor_xcp_function(gcb)
      settings: SourceProductName=Raptor
  raptor_string_length : Raptor_lib/Strings/raptor_string_length  outSize=10
      settings: SourceProductName=Raptor
  raptor_string_printf1 : Raptor_lib/Strings/raptor_string_printf  formatString=' %u %u %f %u %f %.8u\n'
      settings: SourceProductName=Raptor
  raptor_string_toArray : Raptor_lib/Strings/raptor_string_toArray  outSize=100
      settings: SourceProductName=Raptor
  raptor_time1 : Raptor_lib/Triggers/raptor_time  unit=milliseconds
      settings: SourceProductName=Raptor
  wires:
  Sync every 10 Seconds/1(TimeToSync) -> Sync File/Enable
  raptor_string_toArray/1 -> raptor_fileIO_write/2
  raptor_string_printf1/1 -> raptor_string_toArray/1, raptor_string_length/1
  raptor_string/1 -> raptor_string_printf1/1
  raptor_string_length/1 -> raptor_fileIO_write/3
  Data Type Conversion10/1 -> raptor_string_printf1/2
  raptor_fileIO_write/2 -> Terminator1/1
  raptor_fileIO_write/1 -> raptor_fileIO_close/1
  In2/1 -> raptor_fileIO_write/1, Sync File/1(In1)
  Constant/1 -> Add/2
  Add/1 -> raptor_data_write/1
  raptor_data_read1/1 -> Add/1
  Counter Limited/1 -> Data Type Conversion10/1
  raptor_time1/1 -> raptor_string_printf1/7
  In Bus Element5/1 -> Data Type Conversion2/1
  In Bus Element4/1 -> raptor_string_printf1/6
  In Bus Element3/1 -> Data Type Conversion1/1
  In Bus Element2/1 -> raptor_string_printf1/4
  Data Type Conversion1/1 -> raptor_string_printf1/3
  Data Type Conversion2/1 -> raptor_string_printf1/5

== system displayTest/Foreground/Display/Data Logging/Write to Log/Open Existing File ==
  Path : Inport
  Action Port : ActionPort  ActionPortLabel=if(u1)
  File Seek : Subsystem
  Merge : Subsystem
  raptor_fileIO_open1 : Raptor_Datalogging_lib/raptor_fileIO_open  resourceValues=Data|USB|(None)  resource=USB  modeValues=Read Only|Write Only - Overwrite|Read/Write - Update|Read/Write - Overwrite  mode=3
      settings: SourceProductName=Raptor Data Logging
  Handle : Outport  VectorParamsAs1DForOutWhenUnconnected=off
  Sucess : Outport  Port=2  VectorParamsAs1DForOutWhenUnconnected=off
  wires:
  Path/1 -> raptor_fileIO_open1/1
  Merge/1(Handle) -> Handle/1
  Merge/2(Success) -> Sucess/1
  raptor_fileIO_open1/1 -> File Seek/1(Open File Handle)
  raptor_fileIO_open1/2 -> File Seek/2(Open Success)
  File Seek/1(Seek File Handle Success) -> Merge/1(File Handle Success)
  File Seek/2(Seek Success) -> Merge/2(File Open Success)
  File Seek/3(Seek File Handle Failure) -> Merge/3(File Handle Failure)
  File Seek/4(Seek Failure) -> Merge/4(File Open Failure)

== system displayTest/Foreground/Display/Screens/AboutScreen_Create/AboutScreenSwipe ==
  note: This function is called when a swipe action occurs.  The gesture input will
      |  provide the gesture detected:
      |   0 = UP
      |   1 = DOWN
      |   2 = LEFT
      |   3 = RIGHT
  AboutScreenSwipe : TriggerPort  TriggerType=function-call  IsSimulinkFunction=on  FunctionName=AboutScreenSwipe  FunctionVisibility=scoped  VariantControl=Variant  PortDimensions=1
  Constant : Constant  Value=4  OutDataTypeStr=uint8
  Function Caller : FunctionCaller  FunctionPrototype=Screens.Navigation(gesture,curr_screen)  InputArgumentSpecifications=<Enter example>  OutputArgumentSpecifications=<Enter example>
  gesture : ArgIn  OutDataTypeStr=uint8  ArgumentName=gesture
  wires:
  Constant/1 -> Function Caller/2
  gesture/1 -> Function Caller/1
